simulink model "DGL2_01"  (R2020a)
settings: Solver=VariableStepAuto  StartTime=0.0  StopTime=10.0  RelTol=1e-3
values from neighbouring files (symbols this model uses):
  C = [1, 0, 0, 0 ... (first row only)    [bldc_motor.m]    (also in test_simulink.m = 1)
  dUc_dt_0 = 1/C    (= 1)    [test_simulink.m]
  L = 84e-6/2    (= 4.2e-05)    [bldc_motor.m]    (also in test_simulink.m = 10; ueb_simulink_Pendel.m = 10)
  Tau = La/Ra    (= 0.00267462686567)    [test_DC_Motor.m]    (also in test_simulink.m = 10319.9174407; ueb_simulink_ofen.m = 10319.9174407)
  u_in = 1    [test_simulink.m]
  Uc_0 = 0    [test_simulink.m]
  w_2 = 1/(L*C)    (= 1)    [test_simulink.m]
settings Model: Creator=Horst  LastModifiedBy=Horst
settings DataIOCC: ReturnWorkspaceOutputs=off
settings DebuggingCC: ArithmeticOperatorsInVariantConditions=warning
settings SFSimCC: SimUseLocalCustomCode=off  CustomCodeUndefinedFunction=UseInterfaceOnly
settings RTWCC: RTWUseLocalCustomCode=off

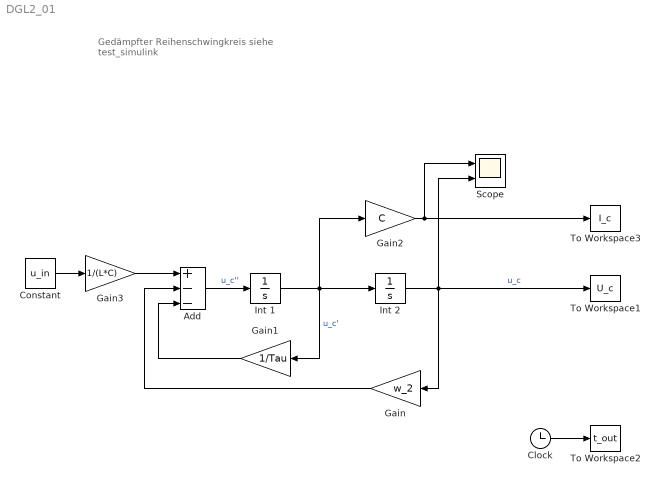
== system DGL2_01 ==
  note: Gedämpfter Reihenschwingkreis
      | siehe test_simulink
  Add : Sum  Inputs=+--
  Clock : Clock
  Constant : Constant  Value=u_in
  Gain : Gain  Gain=w_2
  Gain1 : Gain  Gain=1/Tau
  Gain2 : Gain  Gain=C
  Gain3 : Gain  Gain=1/(L*C)
  Int 1 : Integrator  InitialCondition=dUc_dt_0
  Int 2 : Integrator  InitialCondition=Uc_0
  Scope : Scope  NumInputPorts=2
  To Workspace1 : ToWorkspace  VariableName=U_c  SampleTime=-1
  To Workspace2 : ToWorkspace  VariableName=t_out  SampleTime=-1
  To Workspace3 : ToWorkspace  VariableName=I_c  SampleTime=-1
  wires:
  Int 1/1 -> Gain1/1, Gain2/1, Int 2/1  "u_c'"
  Int 2/1 -> Scope/2, To Workspace1/1, Gain/1  "u_c"
  Clock/1 -> To Workspace2/1
  Add/1 -> Int 1/1  "u_c''"
  Gain2/1 -> Scope/1, To Workspace3/1
  Gain1/1 -> Add/3
  Gain/1 -> Add/2
  Gain3/1 -> Add/1
  Constant/1 -> Gain3/1
